simulink model "Controller"  (R2016a)
settings: Solver=VariableStepAuto  StartTime=0.0  StopTime=10.0  RelTol=1e-3
values from neighbouring files (symbols this model uses):
  K = lqr(A,B,Q,R)    [LQRController.m]    (also in LQRControllerPrevious.m = lqr(sys,Q,R))
undefined symbols (not defined in the file or in its folder): L
settings Model: Creator=VAIO  LastModifiedBy=VAIO

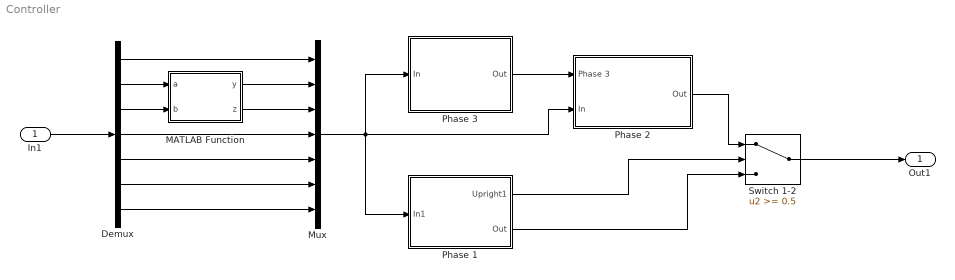
== system Controller ==
  In1 : Inport
  Demux : Demux  Outputs=7
  MATLAB Function : MATLAB Function  TreatAsAtomicUnit=on
  Mux : Mux  Inputs=7
  Phase 1 : Subsystem
  Phase 2 : Subsystem
  Phase 3 : Subsystem
  Switch 1-2 : Switch  Threshold=0.5
  Out1 : Outport
  wires:
  Demux/2 -> MATLAB Function/1(a)
  Demux/3 -> MATLAB Function/2(b)
  Demux/1 -> Mux/1
  MATLAB Function/1(y) -> Mux/2
  MATLAB Function/2(z) -> Mux/3
  Demux/4 -> Mux/4
  Demux/5 -> Mux/5
  Demux/6 -> Mux/6
  Demux/7 -> Mux/7
  In1/1 -> Demux/1
  Mux/1 -> Phase 1/1(In1), Phase 2/2(In), Phase 3/1(In)
  Phase 3/1(Out) -> Phase 2/1(Phase 3)
  Phase 1/1(Upright1) -> Switch 1-2/2
  Phase 1/2(Out) -> Switch 1-2/3
  Phase 2/1(Out) -> Switch 1-2/1
  Switch 1-2/1 -> Out1/1

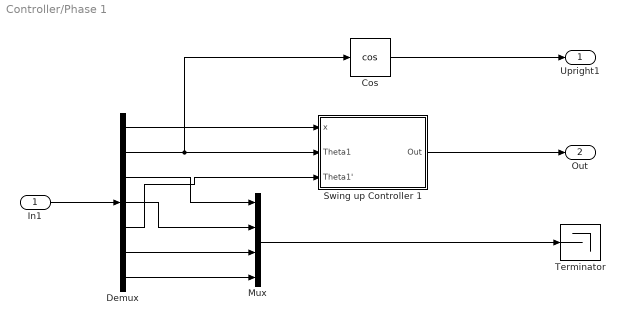
== system Controller/Phase 1 ==
  In1 : Inport
  Cos : Trigonometry  Operator=cos  NumberOfIterations=15
  Demux : Demux  Outputs=7
  Mux : Mux
  Swing up Controller 1 : Subsystem
  Terminator : Terminator
  Upright1 : Outport
  Out : Outport  Port=2
  wires:
  In1/1 -> Demux/1
  Demux/3 -> Mux/1
  Demux/4 -> Mux/2
  Demux/6 -> Mux/3
  Demux/7 -> Mux/4
  Cos/1 -> Upright1/1
  Mux/1 -> Terminator/1
  Demux/1 -> Swing up Controller 1/1(x)
  Swing up Controller 1/1(Out) -> Out/1
  Demux/2 -> Cos/1, Swing up Controller 1/2(Theta1)
  Demux/5 -> Swing up Controller 1/3(Theta1')

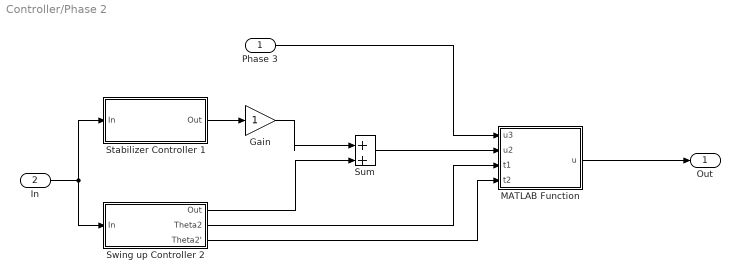
== system Controller/Phase 2 ==
  Phase 3 : Inport
  In : Inport  Port=2
  Gain : Gain
  MATLAB Function : MATLAB Function  TreatAsAtomicUnit=on
  Stabilizer Controller 1 : Subsystem
  Sum : Sum  Inputs=|++
  Swing up Controller 2 : Subsystem
  Out : Outport
  wires:
  MATLAB Function/1(u) -> Out/1
  Gain/1 -> Sum/1
  Sum/1 -> MATLAB Function/2(u2)
  Phase 3/1 -> MATLAB Function/1(u3)
  Stabilizer Controller 1/1(Out) -> Gain/1
  In/1 -> Swing up Controller 2/1(In), Stabilizer Controller 1/1(In)
  Swing up Controller 2/1(Out) -> Sum/2
  Swing up Controller 2/2(Theta2) -> MATLAB Function/3(t1)
  Swing up Controller 2/3(Theta2') -> MATLAB Function/4(t2)

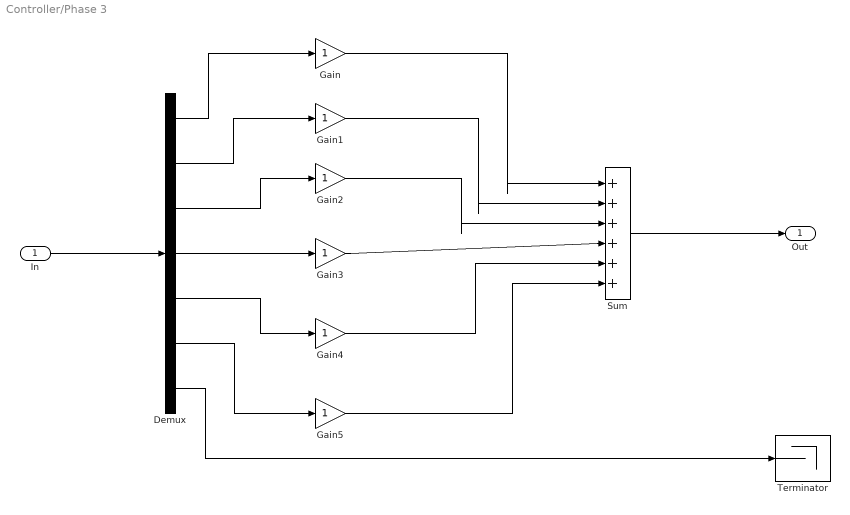
== system Controller/Phase 3 ==
  In : Inport
  Demux : Demux  Outputs=7
  Gain{,1..5} (6 alike) : Gain
  Sum : Sum  Inputs=|++++++
  Terminator : Terminator
  Out : Outport
  wires:
  In/1 -> Demux/1
  Demux/1 -> Gain/1
  Demux/2 -> Gain1/1
  Demux/3 -> Gain2/1
  Demux/4 -> Gain3/1
  Demux/5 -> Gain4/1
  Demux/6 -> Gain5/1
  Sum/1 -> Out/1
  Gain/1 -> Sum/1
  Gain1/1 -> Sum/2
  Gain2/1 -> Sum/3
  Gain3/1 -> Sum/4
  Gain4/1 -> Sum/5
  Gain5/1 -> Sum/6
  Demux/7 -> Terminator/1

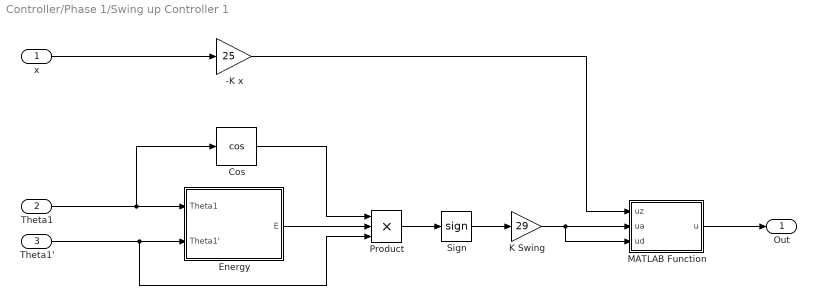
== system Controller/Phase 1/Swing up Controller 1 ==
  x : Inport
  Theta1 : Inport  Port=2  LockScale=on
  Theta1' : Inport  Port=3
  -K x : Gain  Gain=25
  Cos : Trigonometry  Operator=cos  NumberOfIterations=15
  Energy : Subsystem
  K Swing : Gain  Gain=29
  MATLAB Function : MATLAB Function  TreatAsAtomicUnit=on
  Product : Product  Inputs=3
  Sign : Signum
  Out : Outport
  wires:
  MATLAB Function/1(u) -> Out/1
  Sign/1 -> K Swing/1
  K Swing/1 -> MATLAB Function/3(ud), MATLAB Function/2(ua)
  Product/1 -> Sign/1
  x/1 -> -K x/1
  Theta1/1 -> Cos/1, Energy/1(Theta1)
  Theta1'/1 -> Product/3, Energy/2(Theta1')
  Energy/1(E) -> Product/2
  Cos/1 -> Product/1
  -K x/1 -> MATLAB Function/1(uz)

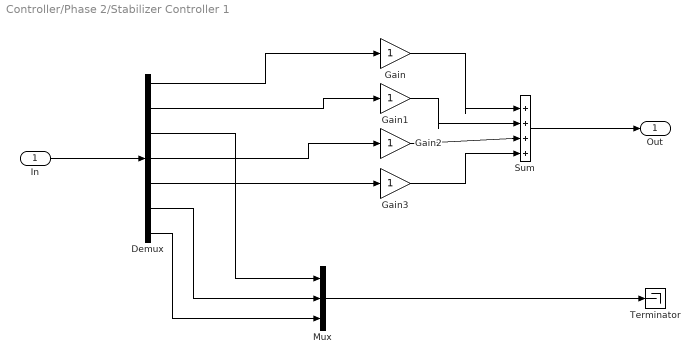
== system Controller/Phase 2/Stabilizer Controller 1 ==
  In : Inport
  Demux : Demux  Outputs=7
  Gain{,1..3} (4 alike) : Gain
  Mux : Mux  Inputs=3
  Sum : Sum  Inputs=|++++
  Terminator : Terminator
  Out : Outport
  wires:
  In/1 -> Demux/1
  Gain/1 -> Sum/1
  Gain1/1 -> Sum/2
  Gain2/1 -> Sum/3
  Gain3/1 -> Sum/4
  Sum/1 -> Out/1
  Demux/1 -> Gain/1
  Demux/2 -> Gain1/1
  Demux/3 -> Mux/1
  Demux/4 -> Gain2/1
  Demux/5 -> Gain3/1
  Demux/6 -> Mux/2
  Demux/7 -> Mux/3
  Mux/1 -> Terminator/1

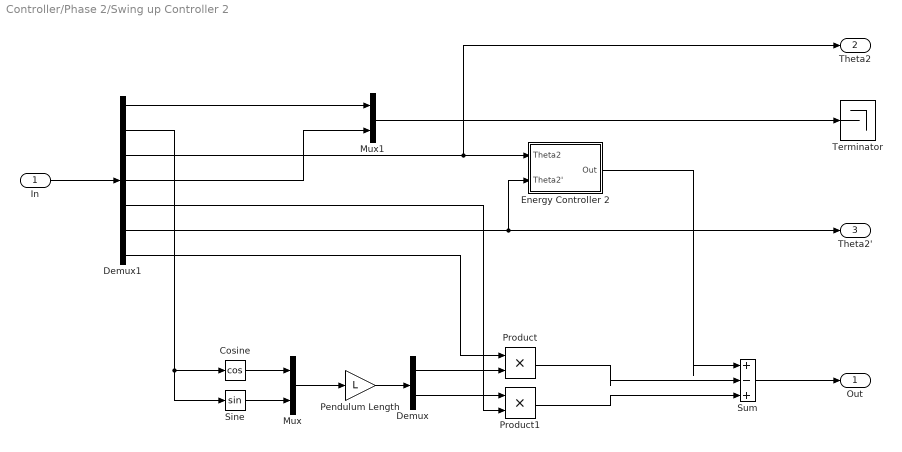
== system Controller/Phase 2/Swing up Controller 2 ==
  In : Inport
  Cosine : Trigonometry  Operator=cos  NumberOfIterations=15
  Demux : Demux  Outputs=2
  Demux1 : Demux  Outputs=7
  Energy Controller 2 : Subsystem
  Mux : Mux  Inputs=2
  Mux1 : Mux  Inputs=2
  Pendulum Length : Gain  Gain=L
  Product : Product
  Product1 : Product
  Sine : Trigonometry  NumberOfIterations=15
  Sum : Sum  Inputs=|+-+
  Terminator : Terminator
  Out : Outport
  Theta2 : Outport  Port=2
  Theta2' : Outport  Port=3
  wires:
  In/1 -> Demux1/1
  Demux1/1 -> Mux1/1
  Demux1/4 -> Mux1/2
  Demux1/3 -> Theta2/1, Energy Controller 2/1(Theta2)
  Product/1 -> Sum/2
  Product1/1 -> Sum/3
  Mux/1 -> Pendulum Length/1
  Pendulum Length/1 -> Demux/1
  Demux/1 -> Product/2
  Demux/2 -> Product1/1
  Demux1/7 -> Product/1
  Demux1/5 -> Product1/2
  Demux1/6 -> Energy Controller 2/2(Theta2'), Theta2'/1
  Sum/1 -> Out/1
  Energy Controller 2/1(Out) -> Sum/1
  Cosine/1 -> Mux/1
  Sine/1 -> Mux/2
  Demux1/2 -> Sine/1, Cosine/1
  Mux1/1 -> Terminator/1

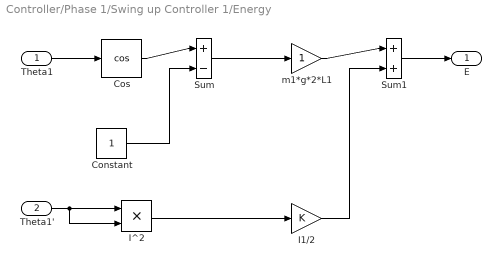
== system Controller/Phase 1/Swing up Controller 1/Energy ==
  Theta1 : Inport
  Theta1' : Inport  Port=2
  Constant : Constant
  Cos : Trigonometry  Operator=cos  NumberOfIterations=15
  I1/2 : Gain  Gain=K
  "I^2 " : Product
  Sum : Sum  Inputs=|+-
  Sum1 : Sum  Inputs=|++
  m1*g*2*L1 : Gain
  E : Outport
  wires:
  Theta1/1 -> Cos/1
  Cos/1 -> Sum/1
  Constant/1 -> Sum/2
  m1*g*2*L1/1 -> Sum1/1
  Sum/1 -> m1*g*2*L1/1
  Sum1/1 -> E/1
  Theta1'/1 -> "I^2 "/2, "I^2 "/1
  "I^2 "/1 -> I1/2/1
  I1/2/1 -> Sum1/2

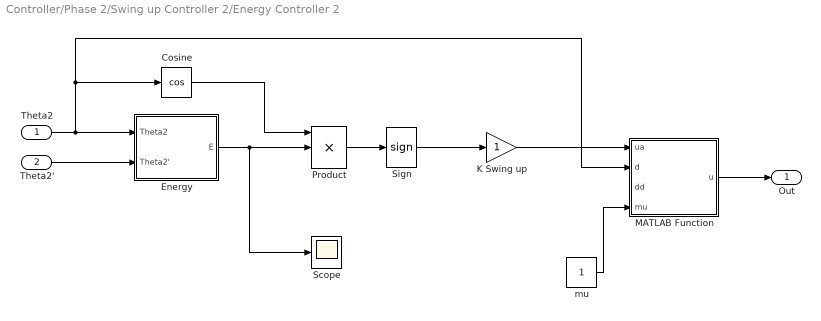
== system Controller/Phase 2/Swing up Controller 2/Energy Controller 2 ==
  Theta2 : Inport
  Theta2' : Inport  Port=2
  Cosine : Trigonometry  Operator=cos  NumberOfIterations=15
  Energy : Subsystem
  K Swing up : Gain
  MATLAB Function : MATLAB Function  TreatAsAtomicUnit=on
  Product : Product  Inputs=3
  Scope : Scope
  Sign : Signum
  mu : Constant
  Out : Outport
  wires:
  MATLAB Function/1(u) -> Out/1
  mu/1 -> MATLAB Function/4(mu)
  K Swing up/1 -> MATLAB Function/1(ua)
  Product/1 -> Sign/1
  Sign/1 -> K Swing up/1
  Energy/1(E) -> Scope/1, Product/2
  Theta2/1 -> Cosine/1, MATLAB Function/2(d), Energy/1(Theta2)
  Theta2'/1 -> Energy/2(Theta2')
  Cosine/1 -> Product/1

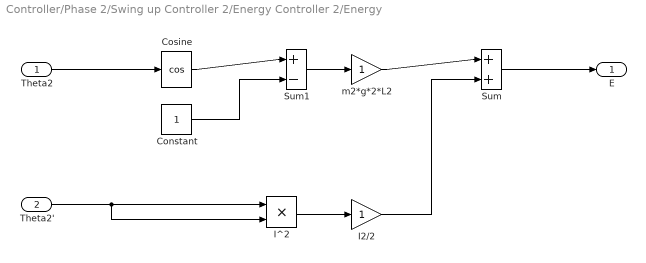
== system Controller/Phase 2/Swing up Controller 2/Energy Controller 2/Energy ==
  Theta2 : Inport
  Theta2' : Inport  Port=2
  Constant : Constant
  Cosine : Trigonometry  Operator=cos  NumberOfIterations=15
  I2/2 : Gain
  I^2 : Product
  Sum : Sum  Inputs=|++
  Sum1 : Sum  Inputs=|+-
  m2*g*2*L2 : Gain
  E : Outport
  wires:
  m2*g*2*L2/1 -> Sum/1
  Sum/1 -> E/1
  I^2/1 -> I2/2/1
  I2/2/1 -> Sum/2
  Sum1/1 -> m2*g*2*L2/1
  Cosine/1 -> Sum1/1
  Constant/1 -> Sum1/2
  Theta2/1 -> Cosine/1
  Theta2'/1 -> I^2/2, I^2/1

== matlab function Controller/Phase 1/Swing up Controller 1/MATLAB Function ==
  data: uz input; u output; ua input; ud input
function u = fcn(uz,ua,ud)

if (abs(ud)>abs(uz))||(sign(ud)==sign(uz))
    u=uz+ua;
elseif (abs(ud)<=abs(uz))&&(sign(ud)~=sign(uz))
    u=ua;
else
    u=0;
end

== matlab function Controller/MATLAB Function ==
  data: a input; y output; b input; z output
function [y,z] = fcn(a,b)

if a>pi
    y=a-2*pi;
elseif a<-pi
    y=a+2*pi;
else
    y=a;
end

if b>pi
    z=b-2*pi;
elseif b<-pi
    z=b+2*pi;
else
    z=b;
end

== matlab function Controller/Phase 2/MATLAB Function ==
  data: u3 input; u output; u2 input; t1 input; t2 input
function u = fcn(u3,u2,t1,t2)

if (cos(t1)>0.97)&&(abs(t2)<=0.5)
    u=u3;
else
    u=u2;
end

% (cos(t1)>0.955)&&(abs(t2)<=0.25)
% cos(t1)>0.97

== matlab function Controller/Phase 2/Swing up Controller 2/Energy Controller 2/MATLAB Function ==
  data: ua input; u output; d input; dd input; mu input
function u = fcn(ua,d,dd,mu)

if ((sin(d)*dd)<0)&&(cos(d)<cos(mu))
    u=ua;
else
    u=0;
end
